simulink model "im_inv_model_mmp"  (R2024b)
settings: Solver=ode1be  StartTime=0.0  StopTime=simlength  FixedStep=tc  MaxStep=tc  EnableMultiTasking=on
undefined symbols (not defined in the file): Adrso_im, alpha_norm, broken_bar_factor, cp, Crso_im, CTRPIFF_CLIP_RELEASE, fPWM_AFE, fPWM_INV, Ibez, iq_lim, kg, ki_i, ki_w, kp_i, kp_w, kw, Ldrso_im, Lm_norm, magnitude, Omega_r_bez, Omega_s_bez, Rr, simlength, speed_m_error_factor, tc, Tcontrol_INV, thermalrise, time_leg_firing_fault_inverter, time_leg_firing_resume_inverter, timeRamp, Tload, ts_afe, ts_inv, Vdc_ref, wref
libraries: fl_lib x41, nesl_utility x40, simulink x2, im_uvw_2_lib x1, threephase_inductor_lib x1, cstblocks x1
(part 1 of 3)
settings Model: SimulationMode=accelerator  Creator=LTNBDA  LastModifiedBy=dbagn
settings SolverCC: ZeroCrossControl=EnableAll  AlgebraicLoopSolver=TrustRegion  AutoInsertRateTranBlk=on
settings DataIOCC: LimitDataPoints=on  MaxDataPoints=1  SaveFormat=Array  SignalLoggingSaveFormat=ModelDataLogs  ReturnWorkspaceOutputs=off
settings OptimizationCC: ReuseModelBlockBuffer=off  ExpressionDepthLimit=2147483647  InitFltsAndDblsToZero=on  LifeSpan=inf
settings DebuggingCC: SaveWithParameterizedLinksMsg=none  UnderspecifiedInitializationDetection=Classic  MergeDetectMultiDrivingBlocksExec=none  SignalResolutionControl=TryResolveAllWithWarning  SolverPrmCheckMsg=warning  MultiTaskDSMMsg=warning  MultiTaskCondExecSysMsg=none  MultiTaskRateTransMsg=warning  FcnCallInpInsideContextMsg=warning  StateNameClashWarn=warning  SFUnexpectedBacktrackingDiag=warning  SFNoUnconditionalDefaultTransitionDiag=warning  SFExecutionAtInitializationDiag=none  ArithmeticOperatorsInVariantConditions=warning
settings HardwareCC: ProdBitPerLong=64  ProdLargestAtomicFloat=None  ProdIntDivRoundTo=Undefined  ProdEndianess=Unspecified  ProdHWDeviceType=Generic->64-bit Embedded Processor (LP64)
settings ModelReferenceCC: EnableRefExpFcnMdlSchedulingChecks=on  PropagateSignalLabelsOutOfModel=off
settings SFSimCC: SimUseLocalCustomCode=off  CustomCodeUndefinedFunction=UseInterfaceOnly
settings SFSimCC: SimCustomHeaderCode=|
  | #include "mavgflt.h"
  | #include "mavgflt_simulink.h"
  | #include "bemf_obsv.h"
  | #include "bemf_obsv_simulink.h"
  | #include "bemf_obsv_load_est.h"
  | #include "bemf_obsv_load_est_simulink.h"
  | #include "bemf_obsv_redu.h"
  | #include "bemf_obsv_redu_simulink.h"
  | #include "bemf_obsv_load_est_redu.h"
  | #include "bemf_obsv_load_est_redu_simulink.h"
  | #include "dqvector_pi.h"
  | #include "dqvector_pi_simulink.h"
  | #include "sv_pwm_simulink.h"
  | #include "sv_pwm.h"
settings SFSimCC: SimUserSources=|
  | "mavgflt_simulink.c"
  | "mavgflt.c"
  | "bemf_obsv_simulink.c"
  | "bemf_obsv.c"
  | "bemf_obsv_load_est_simulink.c"
  | "bemf_obsv_load_est.c"
  | "bemf_obsv_redu_simulink.c"
  | "bemf_obsv_redu.c"
  | "bemf_obsv_load_est_redu_simulink.c"
  | "bemf_obsv_load_est_redu.c"
  | "dqvector_pi.c"
  | "dqvector_pi_simulink.c"
  | "sv_pwm_simulink.c"
  | "sv_pwm.c"
settings SFSimCC: SimUserIncludeDirs=|
  | include
  | src
settings RTWCC: RTWUseLocalCustomCode=off  GPUComputeCapability=3.5
settings CodeAppCC: StateflowObjectComments=on
settings GRTTargetCC: TargetFcnLib=ansi_tfl_tmw.mat  TargetLangStandard=C89/C90 (ANSI)  CombineOutputUpdateFcns=off  GRTInterface=on
settings ConfigComp: CovMetricSettings=dw  CovSaveCumulativeToWorkspaceVar=on  CovSaveSingleToWorkspaceVar=on  CovExternalEMLEnable=off
settings SimscapeCC: SimscapeNormalizeSystem=off

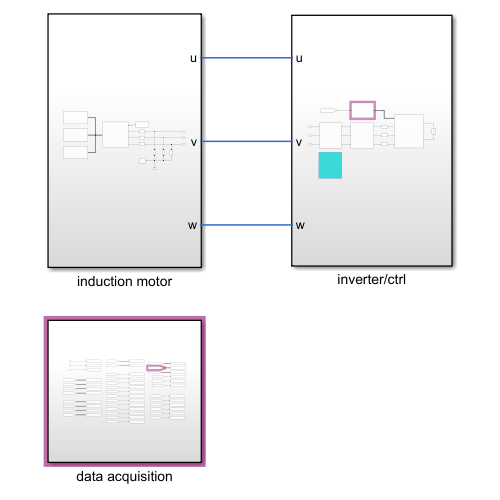
[thumbnail: Simulink's stored preview of the top-level diagram]
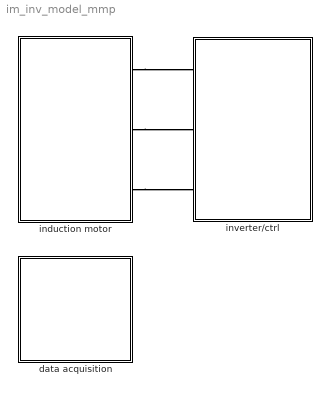
== system im_inv_model_mmp ==
  data acquisition : Subsystem
  induction motor : Subsystem
  inverter/ctrl : Subsystem
  connections:
  induction motor/RConn1 -- inverter/ctrl/LConn1
  induction motor/RConn2 -- inverter/ctrl/LConn2
  induction motor/RConn3 -- inverter/ctrl/LConn3

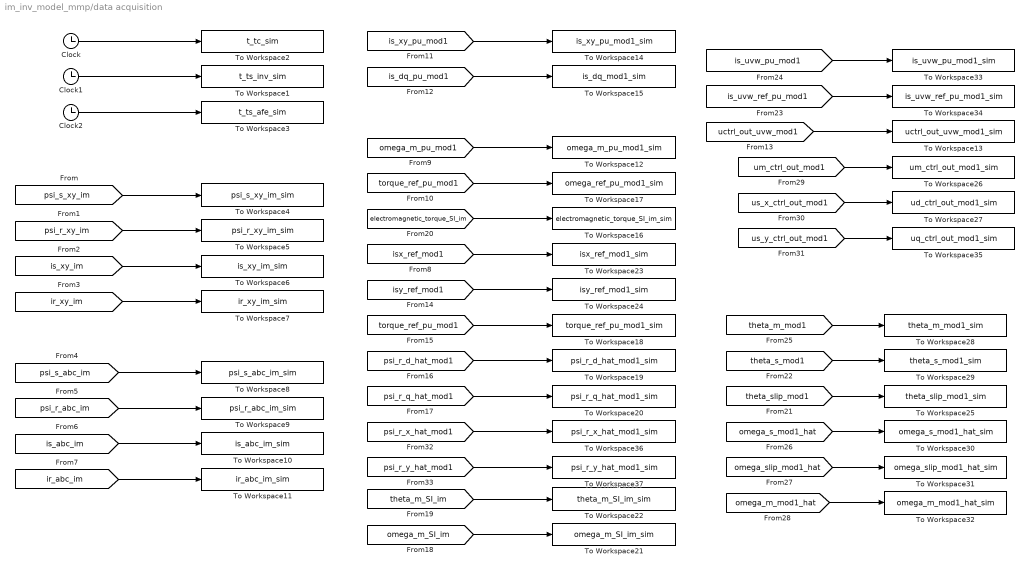
== system im_inv_model_mmp/data acquisition ==
  Clock : Clock
  Clock1 : Clock
  Clock2 : Clock
  To Workspace1 : ToWorkspace  VariableName=t_ts_inv_sim  SampleTime=ts_inv
      settings: MaxDataPoints=Ns_inv
  To Workspace10 : ToWorkspace  VariableName=is_abc_im_sim  SampleTime=tc
      settings: MaxDataPoints=Nc
  To Workspace11 : ToWorkspace  VariableName=ir_abc_im_sim  SampleTime=tc
      settings: MaxDataPoints=Nc
  To Workspace12 : ToWorkspace  VariableName=omega_m_pu_mod1_sim  SampleTime=ts_inv
      settings: MaxDataPoints=Ns_inv
  To Workspace13 : ToWorkspace  VariableName=uctrl_out_uvw_mod1_sim  SampleTime=ts_inv
      settings: MaxDataPoints=Ns_inv
  To Workspace14 : ToWorkspace  VariableName=is_xy_pu_mod1_sim  SampleTime=ts_inv
      settings: MaxDataPoints=Ns_inv
  To Workspace15 : ToWorkspace  VariableName=is_dq_mod1_sim  SampleTime=ts_inv
      settings: MaxDataPoints=Ns_inv
  To Workspace16 : ToWorkspace  VariableName=electromagnetic_torque_SI_im_sim  SampleTime=ts_inv
      settings: MaxDataPoints=Ns_inv
  To Workspace17 : ToWorkspace  VariableName=omega_ref_pu_mod1_sim  SampleTime=ts_inv
      settings: MaxDataPoints=Ns_inv
  To Workspace18 : ToWorkspace  VariableName=torque_ref_pu_mod1_sim  SampleTime=ts_inv
      settings: MaxDataPoints=Ns_inv
  To Workspace19 : ToWorkspace  VariableName=psi_r_d_hat_mod1_sim  SampleTime=ts_inv
      settings: MaxDataPoints=Ns_inv
  To Workspace2 : ToWorkspace  VariableName=t_tc_sim  SampleTime=tc
      settings: MaxDataPoints=Nc
  To Workspace20 : ToWorkspace  VariableName=psi_r_q_hat_mod1_sim  SampleTime=ts_inv
      settings: MaxDataPoints=Ns_inv
  To Workspace21 : ToWorkspace  VariableName=omega_m_SI_im_sim  SampleTime=ts_inv
      settings: MaxDataPoints=Ns_inv
  To Workspace22 : ToWorkspace  VariableName=theta_m_SI_im_sim  SampleTime=ts_inv
      settings: MaxDataPoints=Ns_inv
  To Workspace23 : ToWorkspace  VariableName=isx_ref_mod1_sim  SampleTime=ts_inv
      settings: MaxDataPoints=Ns_inv
  To Workspace24 : ToWorkspace  VariableName=isy_ref_mod1_sim  SampleTime=ts_inv
      settings: MaxDataPoints=Ns_inv
  To Workspace25 : ToWorkspace  VariableName=theta_slip_mod1_sim  SampleTime=ts_inv
      settings: MaxDataPoints=Ns_inv
  To Workspace26 : ToWorkspace  VariableName=um_ctrl_out_mod1_sim  SampleTime=ts_inv
      settings: MaxDataPoints=Ns_afe
  To Workspace27 : ToWorkspace  VariableName=ud_ctrl_out_mod1_sim  SampleTime=ts_inv
      settings: MaxDataPoints=Ns_afe
  To Workspace28 : ToWorkspace  VariableName=theta_m_mod1_sim  SampleTime=ts_inv
      settings: MaxDataPoints=Ns_inv
  To Workspace29 : ToWorkspace  VariableName=theta_s_mod1_sim  SampleTime=ts_inv
      settings: MaxDataPoints=Ns_inv
  To Workspace3 : ToWorkspace  VariableName=t_ts_afe_sim  SampleTime=ts_afe
      settings: MaxDataPoints=Ns_afe
  To Workspace30 : ToWorkspace  VariableName=omega_s_mod1_hat_sim  SampleTime=ts_inv
      settings: MaxDataPoints=Ns_inv
  To Workspace31 : ToWorkspace  VariableName=omega_slip_mod1_hat_sim  SampleTime=ts_inv
      settings: MaxDataPoints=Ns_inv
  To Workspace32 : ToWorkspace  VariableName=omega_m_mod1_hat_sim  SampleTime=ts_inv
      settings: MaxDataPoints=Ns_inv
  To Workspace33 : ToWorkspace  VariableName=is_uvw_pu_mod1_sim  SampleTime=ts_inv
      settings: MaxDataPoints=Ns_afe
  To Workspace34 : ToWorkspace  VariableName=is_uvw_ref_pu_mod1_sim  SampleTime=ts_inv
      settings: MaxDataPoints=Ns_afe
  To Workspace35 : ToWorkspace  VariableName=uq_ctrl_out_mod1_sim  SampleTime=ts_inv
      settings: MaxDataPoints=Ns_afe
  To Workspace36 : ToWorkspace  VariableName=psi_r_x_hat_mod1_sim  SampleTime=ts_inv
      settings: MaxDataPoints=Ns_inv
  To Workspace37 : ToWorkspace  VariableName=psi_r_y_hat_mod1_sim  SampleTime=ts_inv
      settings: MaxDataPoints=Ns_inv
  To Workspace4 : ToWorkspace  VariableName=psi_s_xy_im_sim  SampleTime=tc
      settings: MaxDataPoints=Nc
  To Workspace5 : ToWorkspace  VariableName=psi_r_xy_im_sim  SampleTime=tc
      settings: MaxDataPoints=Nc
  To Workspace6 : ToWorkspace  VariableName=is_xy_im_sim  SampleTime=tc
      settings: MaxDataPoints=Nc
  To Workspace7 : ToWorkspace  VariableName=ir_xy_im_sim  SampleTime=tc
      settings: MaxDataPoints=Nc
  To Workspace8 : ToWorkspace  VariableName=psi_s_abc_im_sim  SampleTime=tc
      settings: MaxDataPoints=Nc
  To Workspace9 : ToWorkspace  VariableName=psi_r_abc_im_sim  SampleTime=tc
      settings: MaxDataPoints=Nc
  wires:
  Clock/1 -> To Workspace2/1
  Clock1/1 -> To Workspace1/1
  Clock2/1 -> To Workspace3/1
  [psi_s_xy_im] -> To Workspace4/1
  [psi_r_xy_im] -> To Workspace5/1
  [is_xy_im] -> To Workspace6/1
  [ir_xy_im] -> To Workspace7/1
  [psi_s_abc_im] -> To Workspace8/1
  [psi_r_abc_im] -> To Workspace9/1
  [is_abc_im] -> To Workspace10/1
  [ir_abc_im] -> To Workspace11/1
  [is_dq_pu_mod1] -> To Workspace15/1
  [uctrl_out_uvw_mod1] -> To Workspace13/1
  [is_xy_pu_mod1] -> To Workspace14/1
  [omega_m_pu_mod1] -> To Workspace12/1
  [electromagnetic_torque_SI_im] -> To Workspace16/1
  [torque_ref_pu_mod1] -> To Workspace17/1
  [omega_m_SI_im] -> To Workspace21/1
  [torque_ref_pu_mod1] -> To Workspace18/1
  [psi_r_d_hat_mod1] -> To Workspace19/1
  [psi_r_q_hat_mod1] -> To Workspace20/1
  [theta_m_SI_im] -> To Workspace22/1
  [isx_ref_mod1] -> To Workspace23/1
  [isy_ref_mod1] -> To Workspace24/1
  [theta_slip_mod1] -> To Workspace25/1
  [theta_m_mod1] -> To Workspace28/1
  [theta_s_mod1] -> To Workspace29/1
  [omega_s_mod1_hat] -> To Workspace30/1
  [omega_slip_mod1_hat] -> To Workspace31/1
  [omega_m_mod1_hat] -> To Workspace32/1
  [is_uvw_pu_mod1] -> To Workspace33/1
  [is_uvw_ref_pu_mod1] -> To Workspace34/1
  [psi_r_x_hat_mod1] -> To Workspace36/1
  [psi_r_y_hat_mod1] -> To Workspace37/1
  [us_x_ctrl_out_mod1] -> To Workspace27/1
  [us_y_ctrl_out_mod1] -> To Workspace35/1
  [um_ctrl_out_mod1] -> To Workspace26/1

== system im_inv_model_mmp/induction motor ==
  Electrical Reference : fl_lib/Electrical/Electrical Elements/Electrical Reference
  Inductor : fl_lib/Electrical/Electrical Elements/Inductor  l=1e-6 H  r=0 Ohm  g=1e-9 1/Ohm  i_specify=off  i_priority=None  i=0 A  i_nominal_specify=off  i_nominal_value=1  i_nominal_unit=A  v_specify=off  v_priority=None  v=0 V  v_nominal_specify=off  v_nominal_value=1  v_nominal_unit=V  i_L_specify=off  i_L_priority=High  i_L=0 A  i_L_nominal_specify=off  i_L_nominal_value=1  i_L_nominal_unit=A
  Inductor1 : fl_lib/Electrical/Electrical Elements/Inductor  l=1e-6 H  r=0 Ohm  g=1e-9 1/Ohm  i_specify=off  i_priority=None  i=0 A  i_nominal_specify=off  i_nominal_value=1  i_nominal_unit=A  v_specify=off  v_priority=None  v=0 V  v_nominal_specify=off  v_nominal_value=1  v_nominal_unit=V  i_L_specify=off  i_L_priority=High  i_L=0 A  i_L_nominal_specify=off  i_L_nominal_value=1  i_L_nominal_unit=A
  Inductor2 : fl_lib/Electrical/Electrical Elements/Inductor  l=1e-6 H  r=0 Ohm  g=1e-9 1/Ohm  i_specify=off  i_priority=None  i=0 A  i_nominal_specify=off  i_nominal_value=1  i_nominal_unit=A  v_specify=off  v_priority=None  v=0 V  v_nominal_specify=off  v_nominal_value=1  v_nominal_unit=V  i_L_specify=off  i_L_priority=High  i_L=0 A  i_L_nominal_specify=off  i_L_nominal_value=1  i_L_nominal_unit=A
  Resistor : fl_lib/Electrical/Electrical Elements/Resistor  R=1e5 Ohm  i_specify=off  i_priority=None  i=0 A  i_nominal_specify=off  i_nominal_value=1  i_nominal_unit=A  v_specify=off  v_priority=None  v=0 V  v_nominal_specify=off  v_nominal_value=1  v_nominal_unit=V
  Resistor1 : fl_lib/Electrical/Electrical Elements/Resistor  R=1e5 Ohm  i_specify=off  i_priority=None  i=0 A  i_nominal_specify=off  i_nominal_value=1  i_nominal_unit=A  v_specify=off  v_priority=None  v=0 V  v_nominal_specify=off  v_nominal_value=1  v_nominal_unit=V
  Resistor2 : fl_lib/Electrical/Electrical Elements/Resistor  R=1e5 Ohm  i_specify=off  i_priority=None  i=0 A  i_nominal_specify=off  i_nominal_value=1  i_nominal_unit=A  v_specify=off  v_priority=None  v=0 V  v_nominal_specify=off  v_nominal_value=1  v_nominal_unit=V
  Solver Configuration : nesl_utility/Solver Configuration  PhysicalDomain=network_engine_domain  SubClassName=solver  LeftPortType=input  RightPortType=generic  Tones=[]  Harmonics=[]  SimulateNoise=off  Profile=off  UseLocalSampling=off  EnableSwitchedLinearOptims=on  FrequencyDomain=off  UseCCode=off  RelTol=0.001  AbsTol=0.001  MinStep=1e-09  ToWorkspace=off  RevertToSquareIcSolve=off  NumHomotopyIterations=100  PhasorMode=off  PhasorModeNumHarmonics=1  ConsistencySolver=NEWTON_XTOL_AFTER_FTOL  IndexReductionMethod=DerivativeReplacement  DoDC=off  ResidualTolerance=1e-09  ConsistencyTolSource=GLOBAL  ConsistencyAbsTol=0.001  ConsistencyRelTol=0.001  ConsistencyTolFactor=0.001  UseLocalSolver=on  LocalSolverChoice=NE_BACKWARD_EULER_ADVANCER  ResolveIndetEquations=on  FunctionEvalNumThread=1  LocalSolverSampleTime=tc  DoFixedCost=on  MaxNonlinIter=3  MaxModeIter=2  ComputeImpulses=off  ImpulseIterations=2  LinearAlgebra=auto  LinearAlgebraNumThread=0  EquationFormulation=NE_TIME_EF  DelaysMemoryBudget=1024  AutomaticFiltering=on  FilteringTimeConstant=0.001  PartitionStorageMethod=AS_NEEDED  PartitionMemoryBudget=1024  PartitionMethod=ROBUST  MultibodyUseLocalSolver=off  MultibodyLocalSolverChoice=ODE1  MultibodyLocalSolverSampleTime=0.001
  control performance evaluation : Subsystem
  induction motor : Subsystem
  load generator : Subsystem
  machine performance evaluation : Subsystem
  mechanical data : Subsystem
  u : PMIOPort  Side=Right
  v : PMIOPort  Port=2  Side=Right
  w : PMIOPort  Port=3  Side=Right
  wires:
  induction motor/1(motor_data) -> control performance evaluation/1(machine_data), machine performance evaluation/1(machine_data), mechanical data/1(machine data)
  load generator/1(torque) -> induction motor/1(torque load)
  connections:
  induction motor/LConn2 -- Inductor1/LConn1
  Inductor/RConn1 -- Resistor/LConn1 -- u/RConn1
  induction motor/LConn3 -- Inductor2/LConn1
  induction motor/LConn1 -- Inductor/LConn1
  v/RConn1 -- Resistor1/LConn1 -- Inductor1/RConn1
  Inductor2/RConn1 -- Resistor2/LConn1 -- w/RConn1
  Resistor/RConn1 -- Solver Configuration/RConn1 -- Resistor2/RConn1 -- Resistor1/RConn1 -- Electrical Reference/LConn1

== system im_inv_model_mmp/inverter//ctrl ==
  DC Voltage Source : fl_lib/Electrical/Electrical Sources/DC Voltage Source  v0=Vdc_ref*1.15 V
  Inductor : fl_lib/Electrical/Electrical Elements/Inductor  l=1e-6 H  r=0 Ohm  g=1e-9 1/Ohm  i_specify=off  i_priority=None  i=0 A  i_nominal_specify=off  i_nominal_value=1  i_nominal_unit=A  v_specify=off  v_priority=None  v=0 V  v_nominal_specify=off  v_nominal_value=1  v_nominal_unit=V  i_L_specify=off  i_L_priority=High  i_L=0 A  i_L_nominal_specify=off  i_L_nominal_value=1  i_L_nominal_unit=A
  Inductor1 : fl_lib/Electrical/Electrical Elements/Inductor  l=1e-6 H  r=0 Ohm  g=1e-9 1/Ohm  i_specify=off  i_priority=None  i=0 A  i_nominal_specify=off  i_nominal_value=1  i_nominal_unit=A  v_specify=off  v_priority=None  v=0 V  v_nominal_specify=off  v_nominal_value=1  v_nominal_unit=V  i_L_specify=off  i_L_priority=High  i_L=0 A  i_L_nominal_specify=off  i_L_nominal_value=1  i_L_nominal_unit=A
  Inductor2 : fl_lib/Electrical/Electrical Elements/Inductor  l=1e-6 H  r=0 Ohm  g=1e-9 1/Ohm  i_specify=off  i_priority=None  i=0 A  i_nominal_specify=off  i_nominal_value=1  i_nominal_unit=A  v_specify=off  v_priority=None  v=0 V  v_nominal_specify=off  v_nominal_value=1  v_nominal_unit=V  i_L_specify=off  i_L_priority=High  i_L=0 A  i_L_nominal_specify=off  i_L_nominal_value=1  i_L_nominal_unit=A
  LFi : threephase_inductor_lib/threephase inductor  Lp=LFi_d H  L0=LFi_0 H  Rp=RLFi_d Ohm  R0=RLFi_0 Ohm  Lls=5e-6 H  uu_1_specify=off  uu_1_priority=None  uu_1=0 V  uu_1_nominal_specify=off  uu_1_nominal_unit=V  uu_1_nominal_value=1  uv_1_specify=off  uv_1_priority=None  uv_1=0 V  uv_1_nominal_specify=off  uv_1_nominal_unit=V  uv_1_nominal_value=1  uw_1_specify=off  uw_1_priority=None  uw_1=0 V  uw_1_nominal_specify=off  uw_1_nominal_unit=V  uw_1_nominal_value=1  uu_2_specify=off  uu_2_priority=None  uu_2=0 V  uu_2_nominal_specify=off  uu_2_nominal_unit=V  uu_2_nominal_value=1  uv_2_specify=off  uv_2_priority=None  uv_2=0 V  uv_2_nominal_specify=off  uv_2_nominal_unit=V  uv_2_nominal_value=1  uw_2_specify=off  uw_2_priority=None  uw_2=0 V  uw_2_nominal_specify=off  uw_2_nominal_unit=V  uw_2_nominal_value=1  iu_specify=off  iu_priority=None  iu=0 A  iu_nominal_specify=off  iu_nominal_unit=A  iu_nominal_value=1  iv_specify=off  iv_priority=None  iv=0 A  iv_nominal_specify=off  iv_nominal_unit=A  iv_nominal_value=1  iw_specify=off  iw_priority=None  iw=0 A  iw_nominal_specify=off  iw_nominal_unit=A  iw_nominal_value=1
      settings: InternalSimscapePortConfiguration="{\"Bottom\":[],\"Left\":[{\"id\":\"up1\",\"label\":\"u1\",\"type\":\"foundation.electrical.electrical\"},{\"id\":\"vp1\",\"label\":\"v1\",\"type\":\"foundation.electrical.electrical\"},{\"id\":\"wp1\",\"label\":\"w1\",\"type\":\"foundation.electrical.electrical\"}],\"Right\":[{\"id\":\"up2\",\"label\":\"u2\",\"type\":\"foundation.electrical.electrical\"},{\"id\":\"vp2\",\"label\":\"v2\",\"type\":\"foundation.electrical.electrical\"},{\"id\":\"wp2\",\"label\":\"w2\",\"type\":\"foundation.electrical.electrical\"}],\"Top\":[]}"
  Subsystem : Subsystem
  im_ctrl : Subsystem
  inverter : Subsystem
  threephase_vi_measures_stack : Subsystem
  u : PMIOPort  Side=Left
  v : PMIOPort  Port=2  Side=Left
  w : PMIOPort  Port=3  Side=Left
  wires:
  [theta_m_mod1] -> im_ctrl/1(theta_m)
  im_ctrl/1(u_ctrl_uvw) -> inverter/1(uctrl_uvw)
  connections:
  LFi/RConn1 -- Inductor/LConn1
  Inductor1/LConn1 -- LFi/RConn2
  LFi/RConn3 -- Inductor2/LConn1
  threephase_vi_measures_stack/LConn1 -- LFi/LConn1
  threephase_vi_measures_stack/LConn2 -- LFi/LConn2
  threephase_vi_measures_stack/LConn3 -- LFi/LConn3
  threephase_vi_measures_stack/RConn3 -- w/RConn1
  threephase_vi_measures_stack/RConn2 -- v/RConn1
  threephase_vi_measures_stack/RConn1 -- u/RConn1
  inverter/LConn1 -- Inductor/RConn1
  inverter/LConn2 -- Inductor1/RConn1
  inverter/LConn3 -- Inductor2/RConn1
  DC Voltage Source/LConn1 -- inverter/RConn1
  DC Voltage Source/RConn1 -- inverter/RConn2

== system im_inv_model_mmp/induction motor/control performance evaluation ==
  machine_data : Inport
  Bus Selector1 : BusSelector  OutputSignals=isu(A),isv(A),isw(A)  OutputAsBus=on
  Bus Selector13 : BusSelector  OutputSignals=psi_s_u(Vs),psi_s_v(Vs),psi_s_w(Vs)  OutputAsBus=on
  Bus Selector14 : BusSelector  OutputSignals=psi_r_u(Vs),psi_r_v(Vs),psi_r_w(Vs)  OutputAsBus=on
  Bus Selector4 : BusSelector  OutputSignals=iru(A),irv(A),irw(A)  OutputAsBus=on
  adc2dq_s_1 : Subsystem
  adc2dq_s_2 : Subsystem
  adc2dq_slip_1 : Subsystem
  adc2dq_slip_2 : Subsystem
  stator/rotor xy currents : Scope  NumInputPorts=2
  stator/rotor xy fluxes : Scope  NumInputPorts=2
  tag scope: ir_abc_im=global, is_abc_im=global, psi_r_abc_im=global, psi_s_abc_im=global
  wires:
  machine_data/1 -> Bus Selector1/1, Bus Selector4/1, Bus Selector14/1, Bus Selector13/1
  Bus Selector13/1 -> [psi_s_abc_im], adc2dq_s_1/1(abc)
  adc2dq_s_1/1(dq) -> stator/rotor xy fluxes/1  "psi_s_dq"
  Bus Selector14/1 -> [psi_r_abc_im], adc2dq_slip_1/1(abc)
  adc2dq_slip_1/1(dq) -> stator/rotor xy fluxes/2  "psi_r_dq"
  adc2dq_slip_2/1(dq) -> stator/rotor xy currents/2  "ir_dq"
  adc2dq_s_2/1(dq) -> stator/rotor xy currents/1  "is_dq"
  Bus Selector1/1 -> [is_abc_im], adc2dq_s_2/1(abc)
  Bus Selector4/1 -> [ir_abc_im], adc2dq_slip_2/1(abc)

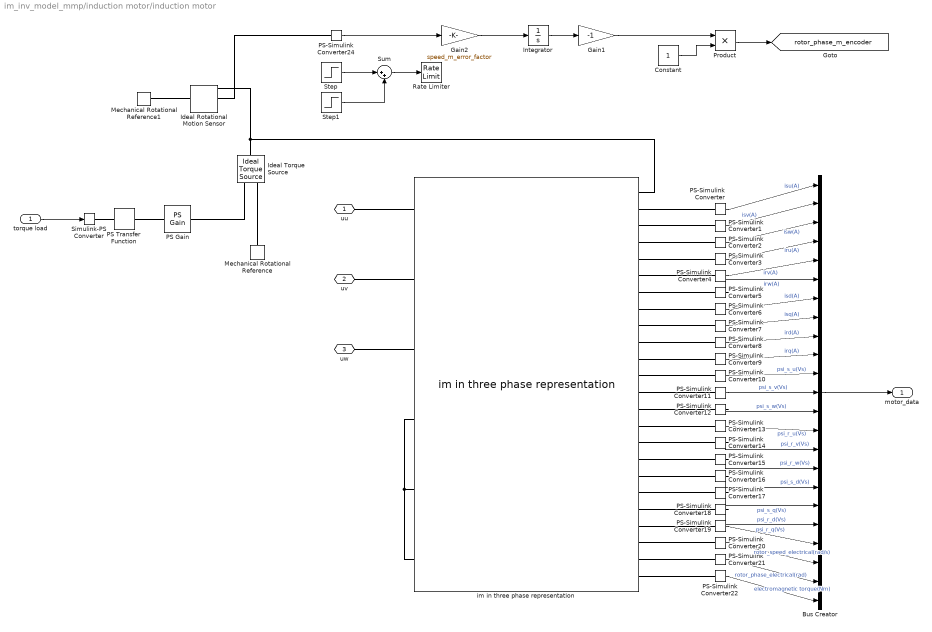
== system im_inv_model_mmp/induction motor/induction motor ==
  torque load : Inport
  Bus Creator : BusCreator  Inputs=23
  Constant : Constant
  Gain1 : Gain  Gain=-1
  Gain2 : Gain  Gain=speed_m_error_factor
  Ideal Rotational Motion Sensor : fl_lib/Mechanical/Mechanical Sensors/Ideal Rotational Motion Sensor  reference=foundation.enum.MeasurementReference.difference  acceleration_port=false  velocity_port=true  position_port=true  wrap_angle=false  offset=0 rad
  Ideal Torque Source : fl_lib/Mechanical/Mechanical Sources/Ideal Torque Source
  Integrator : Integrator
  Mechanical Rotational Reference : fl_lib/Mechanical/Rotational Elements/Mechanical Rotational Reference
  Mechanical Rotational Reference1 : fl_lib/Mechanical/Rotational Elements/Mechanical Rotational Reference
  PS Gain : fl_lib/Physical Signals/Functions/PS Gain  gain=-1
  PS Transfer Function : fl_lib/Physical Signals/Linear Operators/PS Transfer Function  transfer_function_type=foundation.enum.transfer_function_type.lag  T=1/50 s  T1=2 s  T2=1 s  reset_method=foundation.enum.IntegratorResetSpec.None  initial_condition_spec=foundation.enum.IntegratorICSpec.Internal  y0=0 N*m
      settings: InternalSimscapePortConfiguration="{\"Bottom\":[],\"Left\":[{\"id\":\"U\",\"label\":\"\",\"type\":\"input\"}],\"Right\":[{\"id\":\"Y\",\"label\":\"\",\"type\":\"output\"}],\"Top\":[]}"
  PS-Simulink Converter{,1..9} (10 alike) : nesl_utility/PS-Simulink Converter  PhysicalDomain=network_engine_domain  SubClassName=ps_output  LeftPortType=input  RightPortType=output  PseudoPeriodic=off  Frequencies=[]  VectorFormat=1-D array  Unit=A  AffineConversion=off
  PS-Simulink Converter{10..19} (10 alike) : nesl_utility/PS-Simulink Converter  PhysicalDomain=network_engine_domain  SubClassName=ps_output  LeftPortType=input  RightPortType=output  PseudoPeriodic=off  Frequencies=[]  VectorFormat=1-D array  Unit=V*s  AffineConversion=off
  PS-Simulink Converter20 : nesl_utility/PS-Simulink Converter  PhysicalDomain=network_engine_domain  SubClassName=ps_output  LeftPortType=input  RightPortType=output  PseudoPeriodic=off  Frequencies=[]  VectorFormat=1-D array  Unit=rad/s  AffineConversion=off
  PS-Simulink Converter21 : nesl_utility/PS-Simulink Converter  PhysicalDomain=network_engine_domain  SubClassName=ps_output  LeftPortType=input  RightPortType=output  PseudoPeriodic=off  Frequencies=[]  VectorFormat=1-D array  Unit=rad  AffineConversion=off
  PS-Simulink Converter22 : nesl_utility/PS-Simulink Converter  PhysicalDomain=network_engine_domain  SubClassName=ps_output  LeftPortType=input  RightPortType=output  PseudoPeriodic=off  Frequencies=[]  VectorFormat=1-D array  Unit=N*m  AffineConversion=off
  PS-Simulink Converter24 : nesl_utility/PS-Simulink Converter  PhysicalDomain=network_engine_domain  SubClassName=ps_output  LeftPortType=input  RightPortType=output  PseudoPeriodic=off  Frequencies=[]  VectorFormat=1-D array  Unit=rad/s  AffineConversion=off
  Product : Product
  Rate Limiter : RateLimiter  RisingSlewLimit=0.25  FallingSlewLimit=-0.25  SampleTimeMode=inherited
  Simulink-PS Converter : nesl_utility/Simulink-PS Converter  PhysicalDomain=network_engine_domain  SubClassName=ps_input  LeftPortType=input  RightPortType=output  PseudoPeriodic=off  Frequencies=[]  NoiseDistribution=none  NoiseParameters=[]  Unit=N*m  AffineConversion=off  FilteringAndDerivatives=provide  SimscapeFilterOrder=1  InputFilterTimeConstant=0.001  UdotUserProvided=0
  Step : Step  Before=1  After=1.025  SampleTime=0
  Step1 : Step  Time=1.1  After=-0.025  SampleTime=0
  Sum : Sum  Inputs=|++
  im in three phase representation : im_uvw_2_lib/im in three phase representation  Lm=Lm H  Rs=Rs Ohm  Lr=Lr H  Ls=Ls H  Rr=Rr*thermalrise*broken_bar_factor Ohm  Jm=Jrotor kg*m^2  bm=0 N*m*s/rad  pp=cp  omega_m_specify=off  omega_m_priority=None  omega_m=0 rad/s  omega_m_nominal_specify=off  omega_m_nominal_unit=rad/s  omega_m_nominal_value=1  isu_specify=off  isu_priority=None  isu=0 A  isu_nominal_specify=off  isu_nominal_unit=A  isu_nominal_value=1  isv_specify=off  isv_priority=None  isv=0 A  isv_nominal_specify=off  isv_nominal_unit=A  isv_nominal_value=1  isw_specify=off  isw_priority=None  isw=0 A  isw_nominal_specify=off  isw_nominal_unit=A  isw_nominal_value=1  iru_specify=off  iru_priority=None  iru=0 A  iru_nominal_specify=off  iru_nominal_unit=A  iru_nominal_value=1  irv_specify=off  irv_priority=None  irv=0 A  irv_nominal_specify=off  irv_nominal_unit=A  irv_nominal_value=1  irw_specify=off  irw_priority=None  irw=0 A  irw_nominal_specify=off  irw_nominal_unit=A  irw_nominal_value=1  ird_specify=off  ird_priority=None  ird=0 A  ird_nominal_specify=off  ird_nominal_unit=A  ird_nominal_value=1  irq_specify=off  irq_priority=None  irq=0 A  irq_nominal_specify=off  irq_nominal_unit=A  irq_nominal_value=1  isd_specify=off  isd_priority=None  isd=0 A  isd_nominal_specify=off  isd_nominal_unit=A  isd_nominal_value=1  isq_specify=off  isq_priority=None  isq=0 A  isq_nominal_specify=off  isq_nominal_unit=A  isq_nominal_value=1  uu_specify=off  uu_priority=None  uu=0 V  uu_nominal_specify=off  uu_nominal_unit=V  uu_nominal_value=1  uv_specify=off  uv_priority=None  uv=0 V  uv_nominal_specify=off  uv_nominal_unit=V  uv_nominal_value=1  uw_specify=off  uw_priority=None  uw=0 V  uw_nominal_specify=off  uw_nominal_unit=V  uw_nominal_value=1  psi_s_u_specify=off  psi_s_u_priority=None  psi_s_u=0 V*s  psi_s_u_nominal_specify=off  psi_s_u_nominal_unit=V*s  psi_s_u_nominal_value=1  psi_s_v_specify=off  psi_s_v_priority=None  psi_s_v=0 V*s  psi_s_v_nominal_specify=off  psi_s_v_nominal_unit=V*s  psi_s_v_nominal_value=1  psi_s_w_specify=off  psi_s_w_priority=None  psi_s_w=0 V*s  psi_s_w_nominal_specify=off  psi_s_w_nominal_unit=V*s  psi_s_w_nominal_value=1  psi_r_u_specify=off  psi_r_u_priority=None  psi_r_u=0 V*s  psi_r_u_nominal_specify=off  psi_r_u_nominal_unit=V*s  psi_r_u_nominal_value=1  psi_r_v_specify=off  psi_r_v_priority=None  psi_r_v=0 V*s  psi_r_v_nominal_specify=off  psi_r_v_nominal_unit=V*s  psi_r_v_nominal_value=1  psi_r_w_specify=off  psi_r_w_priority=None  psi_r_w=0 V*s  psi_r_w_nominal_specify=off  psi_r_w_nominal_unit=V*s  psi_r_w_nominal_value=1  psi_r_d_specify=off  psi_r_d_priority=None  psi_r_d=0 V*s  psi_r_d_nominal_specify=off  psi_r_d_nominal_unit=V*s  psi_r_d_nominal_value=1  psi_r_q_specify=off  psi_r_q_priority=None  psi_r_q=0 V*s  psi_r_q_nominal_specify=off  psi_r_q_nominal_unit=V*s  psi_r_q_nominal_value=1  psi_s_d_specify=off  psi_s_d_priority=None  psi_s_d=0 V*s  psi_s_d_nominal_specify=off  psi_s_d_nominal_unit=V*s  psi_s_d_nominal_value=1  psi_s_q_specify=off  psi_s_q_priority=None  psi_s_q=0 V*s  psi_s_q_nominal_specify=off  psi_s_q_nominal_unit=V*s  psi_s_q_nominal_value=1  tau_m_specify=off  tau_m_priority=None  tau_m=0 N*m  tau_m_nominal_specify=off  tau_m_nominal_unit=N*m  tau_m_nominal_value=1  tau_l_specify=off  tau_l_priority=None  tau_l=0 N*m  tau_l_nominal_specify=off  tau_l_nominal_unit=N*m  tau_l_nominal_value=1  theta_m_specify=off  theta_m_priority=None  theta_m=0 rad  theta_m_nominal_specify=off  theta_m_nominal_unit=rad  theta_m_nominal_value=1  theta_slip_specify=off  theta_slip_priority=None  theta_slip=0 rad  theta_slip_nominal_specify=off  theta_slip_nominal_unit=rad  theta_slip_nominal_value=1  theta_s_specify=off  theta_s_priority=None  theta_s=0 rad  theta_s_nominal_specify=off  theta_s_nominal_unit=rad  theta_s_nominal_value=1  omega_slip_specify=off  omega_slip_priority=None  omega_slip=0 rad/s  omega_slip_nominal_specify=off  omega_slip_nominal_unit=rad/s  omega_slip_nominal_value=1  omega_s_specify=off  omega_s_priority=None  omega_s=0 rad/s  omega_s_nominal_specify=off  omega_s_nominal_unit=rad/s  omega_s_nominal_value=1
      settings: InternalSimscapePortConfiguration="{\"Bottom\":[],\"Left\":[{\"id\":\"uu_p\",\"label\":\"uu_p\",\"type\":\"foundation.electrical.electrical\"},{\"id\":\"uv_p\",\"label\":\"uv_p\",\"type\":\"foundation.electrical.electrical\"},{\"id\":\"uw_p\",\"label\":\"uw_p\",\"type\":\"foundation.electrical.electrical\"},{\"id\":\"uu_n\",\"label\":\"uu_n\",\"type\":\"foundation.electrical.electrical\"},{\"id\":\"uv_n\",\"label\":\"uv_n\",\"type\":\"foundation.electrical.electrical\"},{\"id\":\"uw_n\",\"label\":\"uw_n\",\"type\":\"foundation.electrical.electrical\"}],\"Right\":[{\"id\":\"S\",\"label\":\"S\",\"type\":\"foundation.mechanical.rotational.rotational\"},{\"id\":\"isu_out\",\"label\":\"isu\",\"type\":\"output\"},{\"id\":\"isv_out\",\"label\":\"isv\",\"type\":\"output\"},{\"id\":\"isw_out\",\"label\":\"isw\",\"type\":\"output\"},{\"id\":\"iru_out\",\"label\":\"iru\",\"type\":\"output\"},{\"id\":\"irv_out\",\"label\":\"irv\",\"type\":\"output\"},{\"id\":\"irw_out\",\"label\":\"irw\",\"type\":\"output\"},{\"id\":\"isd_out\",\"label\":\"isd\",\"type\":\"output\"},{\"id\":\"isq_out\",\"label\":\"isq\",\"type\":\"output\"},{\"id\":\"ird_out\",\"label\":\"ird\",\"type\":\"output\"},{\"id\":\"irq_out\",\"label\":\"irq\",\"type\":\"output\"},{\"id\":\"psi_s_u_out\",\"label\":\"psi_s_u\",\"type\":\"output\"},{\"id\":\"psi_s_v_out\",\"label\":\"psi_s_v\",\"type\":\"output\"},{\"id\":\"psi_s_w_out\",\"label\":\"psi_s_w\",\"type\":\"output\"},{\"id\":\"psi_r_u_out\",\"label\":\"psi_r_u\",\"type\":\"output\"},{\"id\":\"psi_r_v_out\",\"label\":\"psi_r_v\",\"type\":\"output\"},{\"id\":\"psi_r_w_out\",\"label\":\"psi_r_w\",\"type\":\"output\"},{\"id\":\"psi_s_d_out\",\"label\":\"psi_s_d\",\"type\":\"output\"},{\"id\":\"psi_s_q_out\",\"label\":\"psi_s_q\",\"type\":\"output\"},{\"id\":\"psi_r_d_out\",\"label\":\"psi_r_d\",\"type\":\"output\"},{\"id\":\"psi_r_q_out\",\"label\":\"psi_r_q\",\"type\":\"output\"},{\"id\":\"omega_m_out\",\"label\":\"rotor_speed(electrical)\",\"type\":\"output\"},{\"id\":\"theta_m_out\",\"label\":\"rotor_phase(electrical)\",\"type\":\"output\"},{\"id\":\"tau_m_out\",\"label\":\"Electromagnetic torque\",\"type\":\"output\"}],\"Top\":[]}"
  uu : PMIOPort  Side=Left
  uv : PMIOPort  Port=2  Side=Left
  uw : PMIOPort  Port=3  Side=Left
  motor_data : Outport
  tag scope: rotor_phase_m_encoder=global
  wires:
  PS-Simulink Converter/1 -> Bus Creator/1  "isu(A)"
  PS-Simulink Converter1/1 -> Bus Creator/2  "isv(A)"
  PS-Simulink Converter2/1 -> Bus Creator/3  "isw(A)"
  PS-Simulink Converter3/1 -> Bus Creator/4  "iru(A)"
  PS-Simulink Converter4/1 -> Bus Creator/5  "irv(A)"
  PS-Simulink Converter5/1 -> Bus Creator/6  "irw(A)"
  PS-Simulink Converter6/1 -> Bus Creator/7  "isd(A)"
  PS-Simulink Converter7/1 -> Bus Creator/8  "isq(A)"
  PS-Simulink Converter8/1 -> Bus Creator/9  "ird(A)"
  PS-Simulink Converter9/1 -> Bus Creator/10  "irq(A)"
  PS-Simulink Converter10/1 -> Bus Creator/11  "psi_s_u(Vs)"
  PS-Simulink Converter11/1 -> Bus Creator/12  "psi_s_v(Vs)"
  PS-Simulink Converter12/1 -> Bus Creator/13  "psi_s_w(Vs)"
  PS-Simulink Converter13/1 -> Bus Creator/14  "psi_r_u(Vs)"
  PS-Simulink Converter14/1 -> Bus Creator/15  "psi_r_v(Vs)"
  PS-Simulink Converter15/1 -> Bus Creator/16  "psi_r_w(Vs)"
  PS-Simulink Converter16/1 -> Bus Creator/17  "psi_s_d(Vs)"
  PS-Simulink Converter17/1 -> Bus Creator/18  "psi_s_q(Vs)"
  PS-Simulink Converter18/1 -> Bus Creator/19  "psi_r_d(Vs)"
  PS-Simulink Converter19/1 -> Bus Creator/20  "psi_r_q(Vs)"
  PS-Simulink Converter20/1 -> Bus Creator/21  "rotor_speed_electrical(rad/s)"
  PS-Simulink Converter21/1 -> Bus Creator/22  "rotor_phase_electrical(rad)"
  PS-Simulink Converter22/1 -> Bus Creator/23  "electromagnetic torque(Nm)"
  Bus Creator/1 -> motor_data/1
  torque load/1 -> Simulink-PS Converter/1
  Product/1 -> [rotor_phase_m_encoder]
  Step/1 -> Sum/1
  Sum/1 -> Rate Limiter/1
  Gain1/1 -> Product/1
  PS-Simulink Converter24/1 -> Gain2/1
  Integrator/1 -> Gain1/1
  Step1/1 -> Sum/2
  Constant/1 -> Product/2
  Gain2/1 -> Integrator/1
  connections:
  im in three phase representation/LConn1 -- uu/RConn1
  im in three phase representation/LConn3 -- uw/RConn1
  im in three phase representation/LConn2 -- uv/RConn1
  Ideal Torque Source/LConn1 -- Ideal Rotational Motion Sensor/RConn1 -- im in three phase representation/RConn1
  im in three phase representation/LConn4 -- im in three phase representation/LConn6 -- im in three phase representation/LConn5
  PS-Simulink Converter/LConn1 -- im in three phase representation/RConn2
  PS-Simulink Converter1/LConn1 -- im in three phase representation/RConn3
  im in three phase representation/RConn4 -- PS-Simulink Converter2/LConn1
  im in three phase representation/RConn5 -- PS-Simulink Converter3/LConn1
  im in three phase representation/RConn6 -- PS-Simulink Converter4/LConn1
  PS-Simulink Converter5/LConn1 -- im in three phase representation/RConn7
  im in three phase representation/RConn8 -- PS-Simulink Converter6/LConn1
  im in three phase representation/RConn9 -- PS-Simulink Converter7/LConn1
  im in three phase representation/RConn10 -- PS-Simulink Converter8/LConn1
  im in three phase representation/RConn11 -- PS-Simulink Converter9/LConn1
  im in three phase representation/RConn12 -- PS-Simulink Converter10/LConn1
  im in three phase representation/RConn13 -- PS-Simulink Converter11/LConn1
  im in three phase representation/RConn14 -- PS-Simulink Converter12/LConn1
  im in three phase representation/RConn15 -- PS-Simulink Converter13/LConn1
  im in three phase representation/RConn16 -- PS-Simulink Converter14/LConn1
  im in three phase representation/RConn17 -- PS-Simulink Converter15/LConn1
  im in three phase representation/RConn18 -- PS-Simulink Converter16/LConn1
  im in three phase representation/RConn19 -- PS-Simulink Converter17/LConn1
  im in three phase representation/RConn20 -- PS-Simulink Converter18/LConn1
  im in three phase representation/RConn21 -- PS-Simulink Converter19/LConn1
  im in three phase representation/RConn22 -- PS-Simulink Converter20/LConn1
  im in three phase representation/RConn23 -- PS-Simulink Converter21/LConn1
  im in three phase representation/RConn24 -- PS-Simulink Converter22/LConn1
  Mechanical Rotational Reference/LConn1 -- Ideal Torque Source/RConn2
  PS Transfer Function/RConn1 -- PS Gain/LConn1
  Simulink-PS Converter/RConn1 -- PS Transfer Function/LConn1
  PS Gain/RConn1 -- Ideal Torque Source/RConn1
  Ideal Rotational Motion Sensor/RConn2 -- PS-Simulink Converter24/LConn1
  Mechanical Rotational Reference1/LConn1 -- Ideal Rotational Motion Sensor/LConn1

== system im_inv_model_mmp/induction motor/load generator ==
  Gain3 : Gain
  RampSlow : simulink/Sources/Ramp  slope=Tload/timeRamp/simlength*2  start=start_load_ramp  InitialOutput=0
  Saturation : Saturate  UpperLimit=Tload  LowerLimit=-Tload
  Step : Step  After=Tload  SampleTime=0
  torque : Outport
  wires:
  Gain3/1 -> torque/1
  RampSlow/1 -> Saturation/1
  Step/1 -> Gain3/1

== system im_inv_model_mmp/induction motor/machine performance evaluation ==
  machine_data : Inport
  ir_dq : BusSelector  OutputSignals=ird(A),irq(A)  OutputAsBus=on
  is_dq : BusSelector  OutputSignals=isd(A),isq(A)  OutputAsBus=on
  psi_r_dq : BusSelector  OutputSignals=psi_r_d(Vs),psi_r_q(Vs)  OutputAsBus=on
  psi_s_dq : BusSelector  OutputSignals=psi_s_d(Vs),psi_s_q(Vs)  OutputAsBus=on
  rotor/stator currents dq : Scope  NumInputPorts=2
  rotor/stator fluxes xy : Scope  NumInputPorts=2
  tag scope: ir_xy_im=global, is_xy_im=global, psi_r_xy_im=global, psi_s_xy_im=global
  wires:
  machine_data/1 -> psi_r_dq/1, ir_dq/1, is_dq/1, psi_s_dq/1
  psi_r_dq/1 -> [psi_r_xy_im], rotor/stator fluxes xy/1
  psi_s_dq/1 -> [psi_s_xy_im], rotor/stator fluxes xy/2
  ir_dq/1 -> [ir_xy_im], rotor/stator currents dq/1
  is_dq/1 -> [is_xy_im], rotor/stator currents dq/2

== system im_inv_model_mmp/induction motor/mechanical data ==
  machine data : Inport
  Bus Selector1 : BusSelector  OutputSignals=rotor_speed_electrical(rad/s),rotor_phase_electrical(rad),electromagnetic torque(Nm)
  Bus Selector2 : BusSelector  OutputSignals=rotor_phase_electrical(rad)
  Bus Selector3 : BusSelector  OutputSignals=rotor_speed_electrical(rad/s)
  Gain7 : Gain  Gain=1/Omega_s_bez
  Zero-Order Hold1 : ZeroOrderHold  SampleTime=ts_inv
  Zero-Order Hold2 : ZeroOrderHold  SampleTime=ts_inv
  bounder1 : MATLAB Function  TreatAsAtomicUnit=on  SystemSampleTime=ts_inv
  double_integrator_observer_for_im : Subsystem
  encoder_measure : Subsystem
  tag scope: electromagnetic_torque_SI_im=global, omega_m_SI_im=global, omega_m_pu_im=global, omega_m_pu_mod1=global, omega_m_pu_mod2=global, theta_m_SI_im=global, theta_m_im=global, theta_m_mod1=global, theta_m_mod2=global
  wires:
  bounder1/1(y) -> [theta_m_im], [theta_m_mod2], [theta_m_mod1]
  machine data/1 -> Bus Selector1/1, Bus Selector2/1, Bus Selector3/1
  Bus Selector3/1 -> Zero-Order Hold1/1  "<rotor_speed_electrical(rad/s)>"
  Bus Selector2/1 -> Zero-Order Hold2/1  "<rotor_phase_electrical(rad)>"
  Gain7/1 -> [omega_m_pu_mod1], [omega_m_pu_im], [omega_m_pu_mod2]
  Bus Selector1/1 -> [omega_m_SI_im]  "<rotor_speed_electrical(rad/s)>"
  Bus Selector1/3 -> [electromagnetic_torque_SI_im]  "<electromagnetic torque(Nm)>"
  Bus Selector1/2 -> [theta_m_SI_im]  "<rotor_phase_electrical(rad)>"
  double_integrator_observer_for_im/1(omega_hat) -> Gain7/1
  encoder_measure/1(rotor_phase_elec_encoder) -> bounder1/1(u), double_integrator_observer_for_im/1(theta)

== system im_inv_model_mmp/inverter//ctrl/Subsystem ==
  Bus Selector3 : BusSelector  OutputSignals=u_ctrl_u,u_ctrl_v,u_ctrl_w
  Square : Math  Operator=square
  Square Root : Sqrt
  Square1 : Math  Operator=square
  Sum : Sum  Inputs=|++
  abc2dq : Subsystem
  us_x_ctrl_out_mod1/us_y_ctrl_out_mod1 : Scope  NumInputPorts=3
  tag scope: um_ctrl_out_mod1=global, us_x_ctrl_out_mod1=global, us_y_ctrl_out_mod1=global
  wires:
  [us_y_ctrl_out_mod1] -> Square1/1
  Square/1 -> Sum/1
  [uctrl_out_uvw_mod1] -> Bus Selector3/1
  abc2dq/1(d) -> us_x_ctrl_out_mod1/us_y_ctrl_out_mod1/1, [us_x_ctrl_out_mod1]
  Bus Selector3/1 -> abc2dq/1(a)  "<u_ctrl_u>"
  [theta_s_mod1] -> abc2dq/4(wt)
  Bus Selector3/3 -> abc2dq/3(c)  "<u_ctrl_w>"
  Bus Selector3/2 -> abc2dq/2(b)  "<u_ctrl_v>"
  [us_x_ctrl_out_mod1] -> Square/1
  Square1/1 -> Sum/2
  Sum/1 -> Square Root/1
  abc2dq/2(q) -> us_x_ctrl_out_mod1/us_y_ctrl_out_mod1/2, [us_y_ctrl_out_mod1]
  Square Root/1 -> us_x_ctrl_out_mod1/us_y_ctrl_out_mod1/3, [um_ctrl_out_mod1]

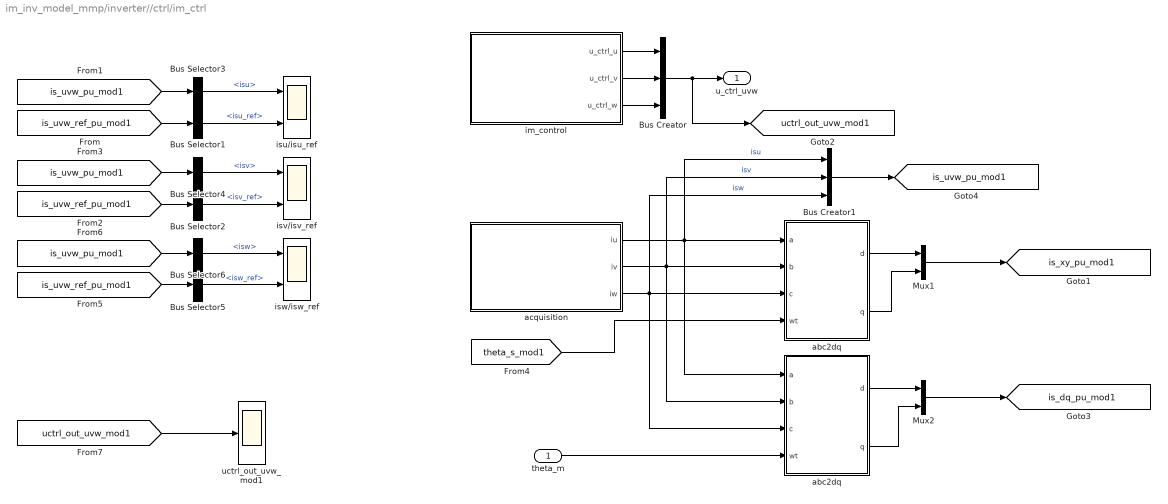
== system im_inv_model_mmp/inverter//ctrl/im_ctrl ==
  theta_m : Inport
  Bus Creator : BusCreator  Inputs=3
  Bus Creator1 : BusCreator  Inputs=3
  Bus Selector1 : BusSelector  OutputSignals=isu_ref
  Bus Selector2 : BusSelector  OutputSignals=isv_ref
  Bus Selector3 : BusSelector  OutputSignals=isu
  Bus Selector4 : BusSelector  OutputSignals=isv
  Bus Selector5 : BusSelector  OutputSignals=isw_ref
  Bus Selector6 : BusSelector  OutputSignals=isw
  Mux1 : Mux  Inputs=2
  Mux2 : Mux  Inputs=2
  abc2dq : Subsystem
  "abc2dq " : Subsystem
  acquisition : Subsystem
  im_control : Subsystem
  isu/isu_ref : Scope  NumInputPorts=2
  isv/isv_ref : Scope  NumInputPorts=2
  isw/isw_ref : Scope  NumInputPorts=2
  uctrl_out_uvw_mod1 : Scope
  u_ctrl_uvw : Outport  VectorParamsAs1DForOutWhenUnconnected=off
  tag scope: is_dq_pu_mod1=global, is_uvw_pu_mod1=global, is_xy_pu_mod1=global, uctrl_out_uvw_mod1=global
  wires:
  Bus Creator/1 -> [uctrl_out_uvw_mod1], u_ctrl_uvw/1
  Mux1/1 -> [is_xy_pu_mod1]
  Mux2/1 -> [is_dq_pu_mod1]
  "abc2dq "/2(q) -> Mux2/2
  "abc2dq "/1(d) -> Mux2/1
  abc2dq/1(d) -> Mux1/1
  abc2dq/2(q) -> Mux1/2
  acquisition/1(iu) -> Bus Creator1/1, abc2dq/1(a), "abc2dq "/1(a)  "isu"
  acquisition/3(iw) -> Bus Creator1/3, abc2dq/3(c), "abc2dq "/3(c)  "isw"
  theta_m/1 -> "abc2dq "/4(wt)
  [theta_s_mod1] -> abc2dq/4(wt)
  Bus Creator1/1 -> [is_uvw_pu_mod1]
  acquisition/2(iv) -> Bus Creator1/2, abc2dq/2(b), "abc2dq "/2(b)  "isv"
  im_control/2(u_ctrl_v) -> Bus Creator/2
  im_control/1(u_ctrl_u) -> Bus Creator/1
  im_control/3(u_ctrl_w) -> Bus Creator/3
  [is_uvw_pu_mod1] -> Bus Selector3/1
  Bus Selector3/1 -> isu/isu_ref/1  "<isu>"
  [is_uvw_ref_pu_mod1] -> Bus Selector1/1
  Bus Selector1/1 -> isu/isu_ref/2  "<isu_ref>"
  Bus Selector2/1 -> isv/isv_ref/2  "<isv_ref>"
  [is_uvw_ref_pu_mod1] -> Bus Selector2/1
  Bus Selector4/1 -> isv/isv_ref/1  "<isv>"
  [is_uvw_pu_mod1] -> Bus Selector4/1
  [is_uvw_pu_mod1] -> Bus Selector6/1
  Bus Selector6/1 -> isw/isw_ref/1  "<isw>"
  [is_uvw_ref_pu_mod1] -> Bus Selector5/1
  Bus Selector5/1 -> isw/isw_ref/2  "<isw_ref>"
  [uctrl_out_uvw_mod1] -> uctrl_out_uvw_mod1/1

== system im_inv_model_mmp/inverter//ctrl/inverter ==
  uctrl_uvw : Inport
  Current Sensor : fl_lib/Electrical/Electrical Sensors/Current Sensor
  PS-Simulink Converter1 : nesl_utility/PS-Simulink Converter  PhysicalDomain=network_engine_domain  SubClassName=ps_output  LeftPortType=input  RightPortType=output  PseudoPeriodic=off  Frequencies=[]  VectorFormat=1-D array  Unit=A  AffineConversion=on
  PS-Simulink Converter4 : nesl_utility/PS-Simulink Converter  PhysicalDomain=network_engine_domain  SubClassName=ps_output  LeftPortType=input  RightPortType=output  PseudoPeriodic=off  Frequencies=[]  VectorFormat=1-D array  Unit=V  AffineConversion=on
  Transfer Fcn : TransferFcn  Denominator=[1e-2 1]
  Voltage Sensor : fl_lib/Electrical/Electrical Sensors/Voltage Sensor
  idc/udc : Scope  NumInputPorts=2
  inverter : Subsystem
  Udc(+) : PMIOPort  Side=Right
  Udc(-) : PMIOPort  Port=2  Side=Right
  us_u : PMIOPort  Port=3  Side=Left
  us_v : PMIOPort  Port=4  Side=Left
  us_w : PMIOPort  Port=5  Side=Left
  wires:
  uctrl_uvw/1 -> inverter/1(uctrl_uvw)
  Transfer Fcn/1 -> idc/udc/1  "idc_flt"
  PS-Simulink Converter1/1 -> Transfer Fcn/1  "idc"
  PS-Simulink Converter4/1 -> idc/udc/2  "udc"
  connections:
  PS-Simulink Converter1/LConn1 -- Current Sensor/RConn1
  Current Sensor/RConn2 -- inverter/RConn1 -- Voltage Sensor/LConn1
  Current Sensor/LConn1 -- Udc(+)/RConn1
  Udc(-)/RConn1 -- inverter/RConn2 -- Voltage Sensor/RConn2
  us_w/RConn1 -- inverter/LConn3
  us_v/RConn1 -- inverter/LConn2
  us_u/RConn1 -- inverter/LConn1
  PS-Simulink Converter4/LConn1 -- Voltage Sensor/RConn1

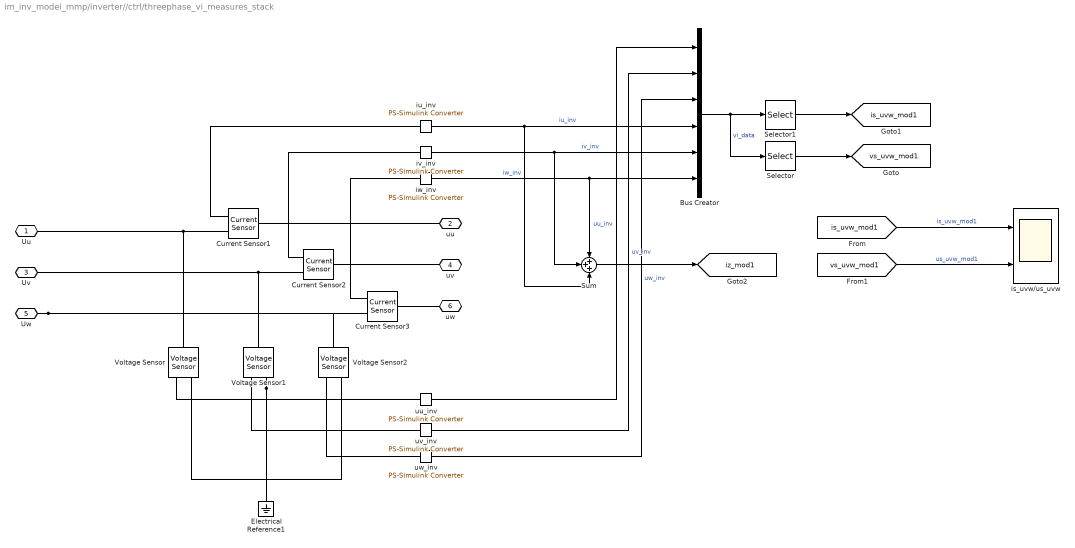
== system im_inv_model_mmp/inverter//ctrl/threephase_vi_measures_stack ==
  Bus Creator : BusCreator  Inputs=6
  Current Sensor1 : fl_lib/Electrical/Electrical Sensors/Current Sensor
  Current Sensor2 : fl_lib/Electrical/Electrical Sensors/Current Sensor
  Current Sensor3 : fl_lib/Electrical/Electrical Sensors/Current Sensor
  Electrical Reference1 : fl_lib/Electrical/Electrical Elements/Electrical Reference
  Selector : Selector  InputPortWidth=6  IndexOptions=Index vector (dialog)  Indices=[1 2 3]  OutputSizes=1
  Selector1 : Selector  InputPortWidth=6  IndexOptions=Index vector (dialog)  Indices=[4 5 6]  OutputSizes=1
  Sum : Sum  Inputs=+++
  Voltage Sensor : fl_lib/Electrical/Electrical Sensors/Voltage Sensor
  Voltage Sensor1 : fl_lib/Electrical/Electrical Sensors/Voltage Sensor
  Voltage Sensor2 : fl_lib/Electrical/Electrical Sensors/Voltage Sensor
  is_uvw/us_uvw : Scope  NumInputPorts=2
  iu_inv : nesl_utility/PS-Simulink Converter  PhysicalDomain=network_engine_domain  SubClassName=ps_output  LeftPortType=input  RightPortType=output  PseudoPeriodic=off  Frequencies=[]  VectorFormat=1-D array  Unit=A  AffineConversion=off
  iv_inv : nesl_utility/PS-Simulink Converter  PhysicalDomain=network_engine_domain  SubClassName=ps_output  LeftPortType=input  RightPortType=output  PseudoPeriodic=off  Frequencies=[]  VectorFormat=1-D array  Unit=A  AffineConversion=off
  iw_inv : nesl_utility/PS-Simulink Converter  PhysicalDomain=network_engine_domain  SubClassName=ps_output  LeftPortType=input  RightPortType=output  PseudoPeriodic=off  Frequencies=[]  VectorFormat=1-D array  Unit=A  AffineConversion=off
  uu_inv : nesl_utility/PS-Simulink Converter  PhysicalDomain=network_engine_domain  SubClassName=ps_output  LeftPortType=input  RightPortType=output  PseudoPeriodic=off  Frequencies=[]  VectorFormat=1-D array  Unit=V  AffineConversion=off
  uv_inv : nesl_utility/PS-Simulink Converter  PhysicalDomain=network_engine_domain  SubClassName=ps_output  LeftPortType=input  RightPortType=output  PseudoPeriodic=off  Frequencies=[]  VectorFormat=1-D array  Unit=V  AffineConversion=off
  uw_inv : nesl_utility/PS-Simulink Converter  PhysicalDomain=network_engine_domain  SubClassName=ps_output  LeftPortType=input  RightPortType=output  PseudoPeriodic=off  Frequencies=[]  VectorFormat=1-D array  Unit=V  AffineConversion=off
  Uu : PMIOPort  Side=Left
  uu : PMIOPort  Port=2  Side=Right
  Uv : PMIOPort  Port=3  Side=Left
  uv : PMIOPort  Port=4  Side=Right
  Uw : PMIOPort  Port=5  Side=Left
  uw : PMIOPort  Port=6  Side=Right
  tag scope: is_uvw_mod1=global, iz_mod1=global, vs_uvw_mod1=global
  wires:
  [vs_uvw_mod1] -> is_uvw/us_uvw/2  "us_uvw_mod1"
  [is_uvw_mod1] -> is_uvw/us_uvw/1  "is_uvw_mod1"
  uw_inv/1 -> Bus Creator/3  "uw_inv"
  uv_inv/1 -> Bus Creator/2  "uv_inv"
  uu_inv/1 -> Bus Creator/1  "uu_inv"
  iw_inv/1 -> Sum/1, Bus Creator/6  "iw_inv"
  iu_inv/1 -> Bus Creator/4, Sum/3  "iu_inv"
  iv_inv/1 -> Bus Creator/5, Sum/2  "iv_inv"
  Selector/1 -> [vs_uvw_mod1]
  Bus Creator/1 -> Selector/1, Selector1/1  "vi_data"
  Selector1/1 -> [is_uvw_mod1]
  Sum/1 -> [iz_mod1]
  connections:
  uw/RConn1 -- Current Sensor3/LConn1
  Voltage Sensor2/RConn1 -- uw_inv/LConn1
  Voltage Sensor/LConn1 -- Current Sensor1/RConn2 -- Uu/RConn1
  Uw/RConn1 -- Current Sensor3/RConn2 -- Voltage Sensor2/LConn1
  Voltage Sensor1/RConn1 -- uv_inv/LConn1
  Voltage Sensor/RConn1 -- uu_inv/LConn1
  Voltage Sensor1/RConn2 -- Voltage Sensor2/RConn2 -- Voltage Sensor/RConn2 -- Electrical Reference1/LConn1
  Voltage Sensor1/LConn1 -- Current Sensor2/RConn2 -- Uv/RConn1
  Current Sensor2/LConn1 -- uv/RConn1
  Current Sensor1/LConn1 -- uu/RConn1
  Current Sensor1/RConn1 -- iu_inv/LConn1
  Current Sensor2/RConn1 -- iv_inv/LConn1
  Current Sensor3/RConn1 -- iw_inv/LConn1

== system im_inv_model_mmp/induction motor/control performance evaluation/adc2dq_s_1 ==
  abc : Inport
  Bus Creator : BusCreator  Inputs=2
  abc2alphabeta : MATLAB Function  TreatAsAtomicUnit=on  SystemSampleTime=tc
  alphabeta2xieta : MATLAB Function  TreatAsAtomicUnit=on  SystemSampleTime=tc
  dq : Outport
  wires:
  abc2alphabeta/1(alpha) -> alphabeta2xieta/1(alpha)  "alpha"
  abc2alphabeta/2(beta) -> alphabeta2xieta/2(beta)  "beta"
  abc/1 -> abc2alphabeta/1(abc)
  [theta_s_mod1] -> alphabeta2xieta/3(theta)
  alphabeta2xieta/1(d) -> Bus Creator/1  "d"
  alphabeta2xieta/2(q) -> Bus Creator/2  "q"
  Bus Creator/1 -> dq/1

== system im_inv_model_mmp/induction motor/control performance evaluation/adc2dq_s_2 ==
  abc : Inport
  Bus Creator : BusCreator  Inputs=2
  abc2alphabeta : MATLAB Function  TreatAsAtomicUnit=on  SystemSampleTime=tc
  alphabeta2xieta : MATLAB Function  TreatAsAtomicUnit=on  SystemSampleTime=tc
  dq : Outport
  wires:
  Bus Creator/1 -> dq/1
  alphabeta2xieta/2(q) -> Bus Creator/2  "q"
  alphabeta2xieta/1(d) -> Bus Creator/1  "d"
  [theta_s_mod1] -> alphabeta2xieta/3(theta)
  abc/1 -> abc2alphabeta/1(abc)
  abc2alphabeta/2(beta) -> alphabeta2xieta/2(beta)  "beta"
  abc2alphabeta/1(alpha) -> alphabeta2xieta/1(alpha)  "alpha"

== system im_inv_model_mmp/induction motor/control performance evaluation/adc2dq_slip_1 ==
  abc : Inport
  Bus Creator : BusCreator  Inputs=2
  abc2alphabeta : MATLAB Function  TreatAsAtomicUnit=on  SystemSampleTime=tc
  alphabeta2xieta : MATLAB Function  TreatAsAtomicUnit=on  SystemSampleTime=tc
  dq : Outport
  wires:
  Bus Creator/1 -> dq/1
  alphabeta2xieta/2(q) -> Bus Creator/2  "q"
  alphabeta2xieta/1(d) -> Bus Creator/1  "d"
  [theta_slip_mod1] -> alphabeta2xieta/3(theta)
  abc/1 -> abc2alphabeta/1(abc)
  abc2alphabeta/2(beta) -> alphabeta2xieta/2(beta)  "beta"
  abc2alphabeta/1(alpha) -> alphabeta2xieta/1(alpha)  "alpha"

== system im_inv_model_mmp/induction motor/control performance evaluation/adc2dq_slip_2 ==
  abc : Inport
  Bus Creator : BusCreator  Inputs=2
  abc2alphabeta : MATLAB Function  TreatAsAtomicUnit=on  SystemSampleTime=tc
  alphabeta2xieta : MATLAB Function  TreatAsAtomicUnit=on  SystemSampleTime=tc
  dq : Outport
  wires:
  abc2alphabeta/1(alpha) -> alphabeta2xieta/1(alpha)  "alpha"
  abc2alphabeta/2(beta) -> alphabeta2xieta/2(beta)  "beta"
  abc/1 -> abc2alphabeta/1(abc)
  [theta_slip_mod1] -> alphabeta2xieta/3(theta)
  alphabeta2xieta/1(d) -> Bus Creator/1  "d"
  alphabeta2xieta/2(q) -> Bus Creator/2  "q"
  Bus Creator/1 -> dq/1

== system im_inv_model_mmp/induction motor/mechanical data/double_integrator_observer_for_im ==
  theta : Inport
  Gain : Gain  Gain=Ldrso_im  Multiplication=Matrix(K*u)
  Gain1 : Gain  Gain=Adrso_im  Multiplication=Matrix(K*u)
  Gain2 : Gain  Gain=Crso_im  Multiplication=Matrix(K*u)
  Selector : Selector  InputPortWidth=2  IndexOptions=Index vector (dialog)  Indices=2  OutputSizes=1
  Sum : Sum  Inputs=-+|
  Sum1 : Sum  Inputs=|++
  Unit Delay : UnitDelay  SampleTime=ts_afe  HasFrameUpgradeWarning=on
  Zero-Order Hold : ZeroOrderHold  SampleTime=ts_afe
  bounder1 : MATLAB Function  TreatAsAtomicUnit=on  SystemSampleTime=ts_afe
  bounder2 : MATLAB Function  TreatAsAtomicUnit=on  SystemSampleTime=ts_afe
  omega_hat : Outport
  wires:
  Gain/1 -> Sum1/1
  Selector/1 -> omega_hat/1
  Gain2/1 -> bounder2/1(u)  "theta_hat"
  Gain1/1 -> Sum1/2
  Sum1/1 -> Unit Delay/1
  Sum/1 -> bounder1/1(u)  "e"
  Unit Delay/1 -> Gain1/1, Selector/1, Gain2/1
  theta/1 -> Zero-Order Hold/1  "theta"
  Zero-Order Hold/1 -> Sum/2  "theta_dsp"
  bounder1/1(y) -> Gain/1  "e_bounded"
  bounder2/1(y) -> Sum/1  "theta_hat_bounded"

== system im_inv_model_mmp/induction motor/mechanical data/encoder_measure ==
  Gain1 : Gain  Gain=cp
  Zero-Order Hold1 : ZeroOrderHold  SampleTime=ts_inv
  bounder2 : MATLAB Function  TreatAsAtomicUnit=on  SystemSampleTime=ts_afe
  rotor_phase_elec_encoder : Outport
  wires:
  [rotor_phase_m_encoder] -> Zero-Order Hold1/1
  Gain1/1 -> bounder2/1(u)
  bounder2/1(y) -> rotor_phase_elec_encoder/1  "e_bounded"
  Zero-Order Hold1/1 -> Gain1/1

== system im_inv_model_mmp/inverter//ctrl/Subsystem/abc2dq ==
  a : Inport
  b : Inport  Port=2
  c : Inport  Port=3
  wt : Inport  Port=4
  abc2alphabeta : Subsystem
  alphabeta2dq : Subsystem
  d : Outport  VectorParamsAs1DForOutWhenUnconnected=off
  q : Outport  Port=2  VectorParamsAs1DForOutWhenUnconnected=off
  wires:
  wt/1 -> alphabeta2dq/3(wt)
  b/1 -> abc2alphabeta/2(b)
  c/1 -> abc2alphabeta/3(c)
  a/1 -> abc2alphabeta/1(a)
  alphabeta2dq/1(d) -> d/1
  alphabeta2dq/2(q) -> q/1
  abc2alphabeta/1("alpha ") -> alphabeta2dq/1(alpha)
  abc2alphabeta/2("beta ") -> alphabeta2dq/2(beta)
